simulink model "FBL_Loop"  (R2020a)
settings: Solver=VariableStepAuto  StartTime=0.0  StopTime=47.7  RelTol=1e-3
libraries: cstblocks x1
settings Model: Creator=apbab  LastModifiedBy=apbab
settings SolverCC: ZeroCrossAlgorithm=Adaptive
settings DebuggingCC: IgnoredZcDiagnostic=none

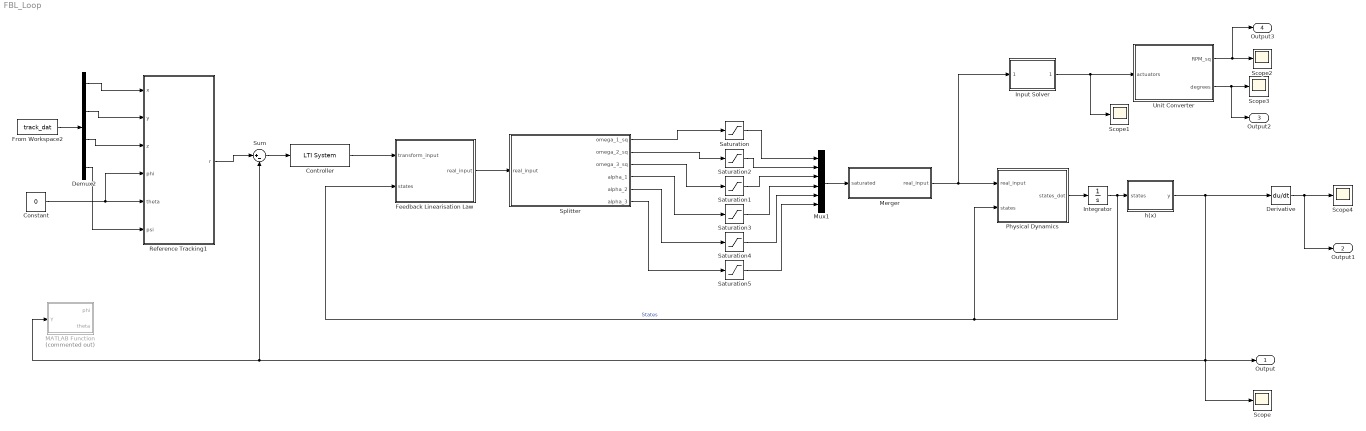
== system FBL_Loop ==
  Constant : Constant  Value=0
  Controller : cstblocks/LTI System  sys=K1  IC=[]
  Demux2 : Demux
  Derivative : Derivative
  Feedback Linearisation Law : MATLAB Function  TreatAsAtomicUnit=on
  From Workspace2 : FromWorkspace  VariableName=track_dat  OutputAfterFinalValue=Holding final value
  Input Solver : MATLAB Function  TreatAsAtomicUnit=on
  Integrator : Integrator
  MATLAB Function : MATLAB Function  Commented=on  TreatAsAtomicUnit=on
  Merger : MATLAB Function  TreatAsAtomicUnit=on
  Mux1 : Mux  Inputs=6
  Physical Dynamics : MATLAB Function  TreatAsAtomicUnit=on
  Reference Tracking1 : MATLAB Function  TreatAsAtomicUnit=on
  Saturation : Saturate  UpperLimit=81e6  LowerLimit=10
  Saturation1 : Saturate  UpperLimit=81e6  LowerLimit=10
  Saturation2 : Saturate  UpperLimit=81e6  LowerLimit=10
  Saturation3 : Saturate  UpperLimit=3  LowerLimit=-3  ZeroCross=off
  Saturation4 : Saturate  UpperLimit=3  LowerLimit=-3  ZeroCross=off
  Saturation5 : Saturate  UpperLimit=3  LowerLimit=-3  ZeroCross=off
  Scope{,1..4} (5 alike) : Scope
  Splitter : MATLAB Function  TreatAsAtomicUnit=on
  Sum : Sum  Inputs=|+-
  Unit Converter : MATLAB Function  TreatAsAtomicUnit=on
  h(x) : MATLAB Function  TreatAsAtomicUnit=on
  Output : Outport
  Output1 : Outport  Port=2
  Output2 : Outport  Port=3
  Output3 : Outport  Port=4
  wires:
  Saturation4/1 -> Mux1/5
  Saturation3/1 -> Mux1/4
  Splitter/6(alpha_3) -> Saturation5/1
  Splitter/2(omega_2_sq) -> Saturation2/1
  Input Solver/1(actuators) -> Scope1/1, Unit Converter/1(actuators)
  Controller/1 -> Feedback Linearisation Law/1(transform_input)
  Derivative/1 -> Output1/1, Scope4/1
  Feedback Linearisation Law/1(real_input) -> Splitter/1(real_input)
  Sum/1 -> Controller/1
  h(x)/1(y) -> Output/1, MATLAB Function/1(Y), Sum/2, Scope/1, Derivative/1
  Merger/1(real_input) -> Input Solver/1(real_input), Physical Dynamics/1(real_input)
  Integrator/1 -> h(x)/1(states), Feedback Linearisation Law/2(states), Physical Dynamics/2(states)  "States"
  Saturation2/1 -> Mux1/2
  Splitter/1(omega_1_sq) -> Saturation/1
  Saturation/1 -> Mux1/1
  Splitter/3(omega_3_sq) -> Saturation1/1
  Splitter/4(alpha_1) -> Saturation3/1
  Splitter/5(alpha_2) -> Saturation4/1
  Saturation1/1 -> Mux1/3
  Saturation5/1 -> Mux1/6
  Physical Dynamics/1(states_dot) -> Integrator/1
  Mux1/1 -> Merger/1(saturated)
  Unit Converter/1(RPM_sq) -> Output3/1, Scope2/1
  Unit Converter/2(degrees) -> Output2/1, Scope3/1
  Reference Tracking1/1(r) -> Sum/1
  Demux2/4 -> Reference Tracking1/6(psi)
  Demux2/2 -> Reference Tracking1/2(y)
  Demux2/1 -> Reference Tracking1/1(x)
  Demux2/3 -> Reference Tracking1/3(z)
  From Workspace2/1 -> Demux2/1
  Constant/1 -> Reference Tracking1/4(phi), Reference Tracking1/5(theta)

== matlab function FBL_Loop/Feedback Linearisation Law ==
  data: transform_input input; states input; real_input output
% This function applies classical feedback linearisation law



% Inputs:
%   transform_input: This is the transformed input v, whose value has been
%                    defined by the main controller.It is a 6x1 vector.
%   states:          This is a 12x1 vector of numerical values for all 12 
%                    states,obtained from the output of the FBL loop

% Output:
%   real_input: The 'true' input of the system, defined as u = rho, where
%               rho is a 6x1 vector of with terms of form 
%               omega_i^2*sin(alpha_i) and omega_i^2*cos(alpha_i)

function real_input = fcn(transform_input,states)

% Initialise dimension of output vector
real_input = zeros(6,1);

% Declare RFBLblock as an extrinsic function
coder.extrinsic('FBLblock')

% Apply RFBLblock function for numerical result
real_input = FBLblock(transform_input,states);

end

== matlab function FBL_Loop/Physical Dynamics ==
  data: real_input input; states input; states_dot output
% This function applies the nonlinear dynamics equations to obtain the
% time-derivatives of the states

% Inputs:
%   real_input: The 'true' input of the system, defined as u = rho, where
%               rho is a 6x1 vector with terms of form 
%               omega_i^2*sin(alpha_i) and omega_i^2*cos(alpha_i). Obtained
%               from FBL law block, and expressed as numerical values
%   states:     This is a 12x1 vector of numerical values for all 12  
%               states, obtained from the output of the FBL loop

% Output:
%   states_dot: 12x1 vector of numerical values for the time derivatives of
%               all 12 states

function states_dot = fcn(real_input,states)

% Initialise dimension of output vector
states_dot = zeros(12,1);

% Declare dynamicsblock as an extrinsic function
coder.extrinsic('dynamicsblock')

% Apply dynamicsblock function for numerical result
states_dot = dynamicsblock(real_input,states);


end

== matlab function FBL_Loop/h(x) ==
  data: states input; y output
function y = fcn(states)

y = [states(7);
          states(8);
          states(9);
          states(10);
          states(11);
          states(12)];

== matlab function FBL_Loop/Input Solver ==
  data: real_input input; actuators output
function actuators = fcn(real_input)

alpha_1 = atan(real_input(1)/real_input(4));
alpha_2 = atan(real_input(2)/real_input(5));
alpha_3 = atan(real_input(3)/real_input(6));

% Currently solving for omega^2 so that we always get real values.
% The goal is for omega^2 to never be negative!!!
omega_1 = ((real_input(1)/sin(alpha_1)));
omega_2 = ((real_input(2)/sin(alpha_2)));
omega_3 = ((real_input(3)/sin(alpha_3)));


actuators = [omega_1, omega_2, omega_3, alpha_1, alpha_2, alpha_3]';
end

== matlab function FBL_Loop/Splitter ==
  data: real_input input; omega_1_sq output; omega_2_sq output; omega_3_sq output; alpha_1 output; alpha_2 output; alpha_3 output
% Splits real input into tilt angles and omega^2 values in order to apply
% saturation limits

function [omega_1_sq,omega_2_sq,omega_3_sq,alpha_1,...
    alpha_2,alpha_3] = fcn(real_input)

alpha_1 = atan(real_input(1)/real_input(4));
alpha_2 = atan(real_input(2)/real_input(5));
alpha_3 = atan(real_input(3)/real_input(6));

omega_1_sq = ((real_input(1)/sin(alpha_1)));
omega_2_sq = ((real_input(2)/sin(alpha_2)));
omega_3_sq = ((real_input(3)/sin(alpha_3)));



end

== matlab function FBL_Loop/Merger ==
  data: saturated input; real_input output
% Merges back together the inputs after saturation limits applied


function real_input = fcn(saturated)

real_input = [saturated(1)*sin(saturated(4));
              saturated(2)*sin(saturated(5));
              saturated(3)*sin(saturated(6));
              saturated(1)*cos(saturated(4));
              saturated(2)*cos(saturated(5));
              saturated(3)*cos(saturated(6))];

== matlab function FBL_Loop/Unit Converter ==
  data: actuators input; RPM_sq output; degrees output
% Converts rotor speeds to RPM and angles to degrees

function [RPM_sq,degrees] = fcn(actuators)

RPM_sq = actuators(1:3)*(30/pi)^2;
degrees = actuators(4:6)*180/pi;

== matlab function FBL_Loop/Reference Tracking1 ==
  data: x input; y input; z input; phi input; theta input; r output; psi input
function  r = fcn(x,y,z,phi,theta,psi)
r = zeros(6,1);
% reference output
r(1) = phi;
r(2) = theta;
r(3) = psi;
r(4) = x;
r(5) = y;
r(6) = z;

== matlab function FBL_Loop/MATLAB Function ==
  data: Y input; phi output; theta output
function [phi,theta] = fcn(Y)

phi = Y(1);
theta = Y(2);
